simulink model "ForwardBackwards_Euler_Model"  (R2019b)
settings: Solver=ode8  StartTime=0.0  StopTime=20  FixedStep=dT  RelTol=1e-3
values from neighbouring files (symbols this model uses):
  dT = [1 1/8 1/80 1/600]    [ForwardBackwards_Euler_Script.m]
undefined symbols (not defined in the file or in its folder): DiscIntNeverNeededParam, k
libraries: simulink x4
settings Model: Creator=crbon  LastModifiedBy=crbon

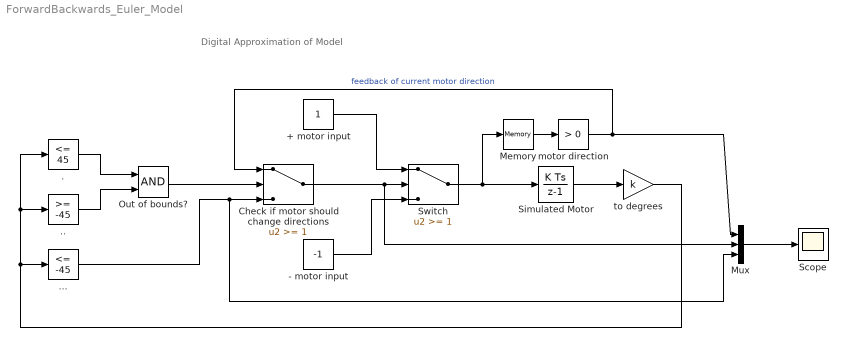
== system ForwardBackwards_Euler_Model ==
  note: Digital Approximation of Model
  + motor input : Constant
  - motor input : Constant  Value=-1
  . : simulink/Logic and Bit Operations/Compare To Constant  relop=<=  const=45  OutDataTypeStr=boolean
  ".. " : simulink/Logic and Bit Operations/Compare To Constant  relop=>=  const=-45  OutDataTypeStr=boolean
  "... " : simulink/Logic and Bit Operations/Compare To Constant  relop=<=  const=-45  OutDataTypeStr=boolean
  Check if motor should change directions : Switch  Threshold=1
  Memory : Memory
  Mux : Mux  Inputs=3
  Out of bounds? : Logic  AllPortsSameDT=off  OutDataTypeStr=boolean
  Scope : Scope
  Simulated Motor : DiscreteIntegrator  SampleTime=dT  ICPrevOutput=DiscIntNeverNeededParam  ICPrevScaledInput=DiscIntNeverNeededParam
  Switch : Switch  Threshold=1
  motor direction : simulink/Logic and Bit Operations/Compare To Constant  relop=>  const=0  OutDataTypeStr=boolean
  to degrees : Gain  Gain=k
  wires:
  + motor input/1 -> Switch/1
  - motor input/1 -> Switch/3
  ".. "/1 -> Out of bounds?/2
  ./1 -> Out of bounds?/1
  Memory/1 -> motor direction/1
  motor direction/1 -> Check if motor should change directions/1, Mux/1  "feedback of current motor direction"
  Simulated Motor/1 -> to degrees/1
  Switch/1 -> Simulated Motor/1, Memory/1
  to degrees/1 -> ./1, ".. "/1, "... "/1
  Out of bounds?/1 -> Check if motor should change directions/2
  Check if motor should change directions/1 -> Mux/2, Switch/2
  Mux/1 -> Scope/1
  "... "/1 -> Mux/3, Check if motor should change directions/3
